simulink library "threeDofDynamics"  (R2020a)
settings: Solver=VariableStepAuto  StartTime=0.0  StopTime=10.0  RelTol=1e-3
libraries: rotationFromGroundToTangent x1
settings Model: Creator=Ayaz  LastModifiedBy=Ayaz

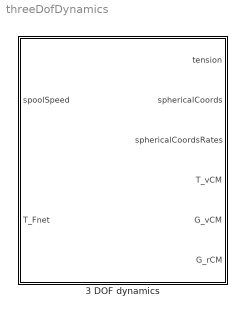
== system threeDofDynamics ==
  3 DOF dynamics : Subsystem  mask{mass=0, init_radius=0, init_azim=0, init_elev=0, init_dAzim=0, init_dElev=0}
      mask prompts: mass "Kite mass [kg]"; init_radius "Initial sphere radius [m]"; init_azim "Initial azimuth angle [rad]"; init_elev "Initial elevation angle [rad]"; init_dAzim "Initial azimuth angle rate [rad/s]"; init_dElev "Initial elevation angle rate [rad/s]"

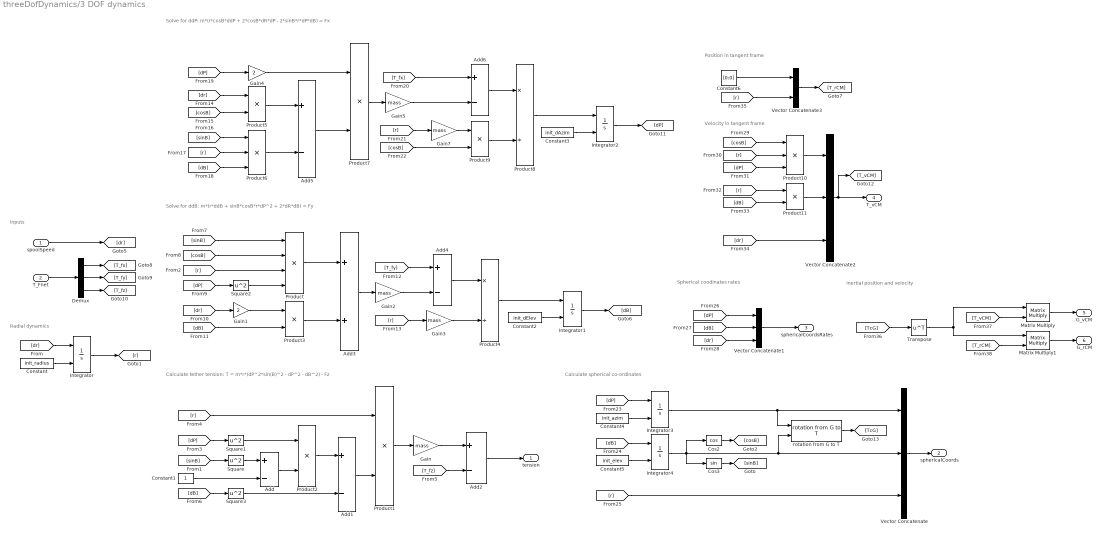
== system threeDofDynamics/3 DOF dynamics ==
  note: inputs
  note: Inertial position and velocity
  note: Position in tangent frame
  note: Velocity in tangent frame
  note: Spherical coodinates rates
  note: Calculate spherical co-ordinates
  note: Solve for ddP: m*(r*cosB*ddP + 2*cosB*dR*dP - 2*sinB*r*dP*dB) = Fx
  note: Solve for ddB: m*(r*ddB + sinB*cosB*r*dP^2 + 2*dR*dB) = Fy
  note: Calculate tether tension: T = m*r*(dP^2*sin(B)^2 - dP^2 - dB^2) - Fz
  note: Radial dynamics
  spoolSpeed : Inport
  T_Fnet : Inport  Port=2
  Add{,1..2,4..6} (6 alike) : Sum  Inputs=+-
  Add3 : Sum
  Constant : Constant  Value=init_radius  VectorParams1D=off
  Constant1 : Constant
  Constant2 : Constant  Value=init_dElev  VectorParams1D=off
  Constant3 : Constant  Value=init_dAzim  VectorParams1D=off
  Constant4 : Constant  Value=init_azim  VectorParams1D=off
  Constant5 : Constant  Value=init_elev  VectorParams1D=off
  Constant6 : Constant  Value=[0;0]  VectorParams1D=off
  Cos2 : Trigonometry  Operator=cos
  Cos3 : Trigonometry
  Demux : Demux  Outputs=3
  Gain{,2..3,5,7} (5 alike) : Gain  Gain=mass
  Gain1 : Gain  Gain=2
  Gain4 : Gain  Gain=2
  Integrator{,1..4} (5 alike) : Integrator  InitialConditionSource=external
  Matrix Multiply : Product  Multiplication=Matrix(*)
  Matrix Multiply1 : Product  Multiplication=Matrix(*)
  Product : Product  Inputs=4
  Product{1..3,5,7,9,11} (7 alike) : Product
  Product10 : Product  Inputs=3
  Product4 : Product  Inputs=*/
  Product6 : Product  Inputs=3
  Product8 : Product  Inputs=*/
  Square{,1..3} (4 alike) : Math  Operator=square  SaturateOnIntegerOverflow=on
  Transpose : Math  Operator=transpose  SaturateOnIntegerOverflow=on
  Vector Concatenate : Concatenate  NumInputs=3
  Vector Concatenate1 : Concatenate  NumInputs=3
  Vector Concatenate2 : Concatenate  NumInputs=3
  Vector Concatenate3 : Concatenate
  rotation from G to T : rotationFromGroundToTangent/rotation from G to T  SystemSampleTime=-1  Latency=0  AutoFrameSizeCalculation=off
  tension : Outport  PortDimensions=[1,1]
  sphericalCoords : Outport  Port=2  PortDimensions=[3,1]
  sphericalCoordsRates : Outport  Port=3  PortDimensions=[3,1]
  T_vCM : Outport  Port=4  PortDimensions=[3,1]
  G_vCM : Outport  Port=5  PortDimensions=[3,1]
  G_rCM : Outport  Port=6
  wires:
  Constant/1 -> Integrator/2
  spoolSpeed/1 -> [dr]
  [dr] -> Integrator/1
  Integrator/1 -> [r]
  [sinB] -> Square/1
  Square/1 -> Add/1
  [dP] -> Square1/1
  [r] -> Product1/1
  Constant1/1 -> Add/2
  Add/1 -> Product2/2
  Square1/1 -> Product2/1
  [dB] -> Square3/1
  Product2/1 -> Add1/1
  Square3/1 -> Add1/2
  Add1/1 -> Product1/2
  T_Fnet/1 -> Demux/1
  Demux/1 -> [T_fx]
  Demux/2 -> [T_fy]
  Demux/3 -> [T_fz]
  Product1/1 -> Gain/1
  Gain/1 -> Add2/1
  [T_fz] -> Add2/2
  Add2/1 -> tension/1
  Square2/1 -> Product/4
  [dP] -> Square2/1
  [sinB] -> Product/1
  [cosB] -> Product/2
  [r] -> Product/3
  Product/1 -> Add3/1
  [dr] -> Gain1/1
  Gain1/1 -> Product3/1
  [dB] -> Product3/2
  Product3/1 -> Add3/2
  Add3/1 -> Gain2/1
  [T_fy] -> Add4/1
  Gain2/1 -> Add4/2
  Add4/1 -> Product4/1
  Gain3/1 -> Product4/2
  [r] -> Gain3/1
  Product4/1 -> Integrator1/1
  Constant2/1 -> Integrator1/2
  Integrator1/1 -> [dB]
  [dr] -> Product5/1
  [cosB] -> Product5/2
  Product5/1 -> Add5/1
  [sinB] -> Product6/1
  [r] -> Product6/2
  [dB] -> Product6/3
  Product6/1 -> Add5/2
  Add5/1 -> Product7/2
  [dP] -> Gain4/1
  Gain4/1 -> Product7/1
  Product7/1 -> Gain5/1
  [T_fx] -> Add6/1
  Gain5/1 -> Add6/2
  Add6/1 -> Product8/1
  [r] -> Gain7/1
  Gain7/1 -> Product9/1
  [cosB] -> Product9/2
  Product9/1 -> Product8/2
  Integrator2/1 -> [dP]
  Constant3/1 -> Integrator2/2
  Product8/1 -> Integrator2/1
  [dP] -> Integrator3/1
  Constant4/1 -> Integrator3/2
  [dB] -> Integrator4/1
  Constant5/1 -> Integrator4/2
  Integrator3/1 -> rotation from G to T/1, Vector Concatenate/1
  Integrator4/1 -> Cos3/1, Cos2/1, rotation from G to T/2, Vector Concatenate/2
  [r] -> Vector Concatenate/3
  Vector Concatenate/1 -> sphericalCoords/1
  Cos3/1 -> [sinB]
  Cos2/1 -> [cosB]
  [dP] -> Vector Concatenate1/1
  [dB] -> Vector Concatenate1/2
  [dr] -> Vector Concatenate1/3
  Vector Concatenate1/1 -> sphericalCoordsRates/1
  [cosB] -> Product10/1
  [r] -> Product10/2
  [dP] -> Product10/3
  [r] -> Product11/1
  [dB] -> Product11/2
  Product10/1 -> Vector Concatenate2/1
  Product11/1 -> Vector Concatenate2/2
  [dr] -> Vector Concatenate2/3
  Vector Concatenate2/1 -> [T_vCM], T_vCM/1
  Constant6/1 -> Vector Concatenate3/1
  [r] -> Vector Concatenate3/2
  Vector Concatenate3/1 -> [T_rCM]
  rotation from G to T/1 -> [TcG]
  [TcG] -> Transpose/1
  Transpose/1 -> Matrix Multiply1/1, Matrix Multiply/1
  [T_vCM] -> Matrix Multiply/2
  [T_rCM] -> Matrix Multiply1/2
  Matrix Multiply/1 -> G_vCM/1
  Matrix Multiply1/1 -> G_rCM/1
